simulink subsystem "YawController_SubSystem"  (R2021a)
settings: Solver=VariableStepAuto  StartTime=0.0  StopTime=10.0  RelTol=1e-3
undefined symbols (not defined in the file): DiscIntNeverNeededParam, drv, Ts, yaw_Ki, yaw_Kp
settings Model: Creator=utente-A  LastModifiedBy=utente-A

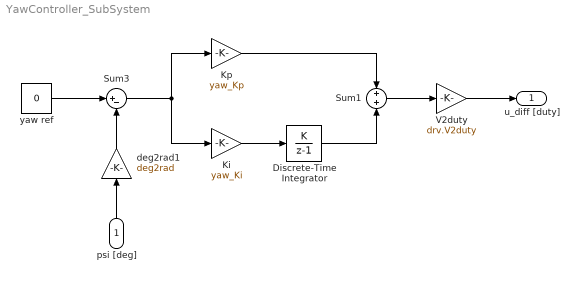
== system YawController_SubSystem ==
  psi [deg] : Inport
  Discrete-Time Integrator : DiscreteIntegrator  IntegratorMethod=Accumulation: Forward Euler  SampleTime=Ts  ICPrevOutput=DiscIntNeverNeededParam  ICPrevScaledInput=DiscIntNeverNeededParam
  Ki : Gain  Gain=yaw_Ki
  Kp : Gain  Gain=yaw_Kp
  Sum1 : Sum
  Sum3 : Sum  Inputs=|+-
  V2duty : Gain  Gain=drv.V2duty
  deg2rad1 : Gain  Gain=deg2rad
  yaw ref : Constant  Value=0
  u_diff [duty] : Outport
  wires:
  Sum3/1 -> Kp/1, Ki/1
  psi [deg]/1 -> deg2rad1/1
  deg2rad1/1 -> Sum3/2
  Ki/1 -> Discrete-Time Integrator/1
  Kp/1 -> Sum1/1
  Discrete-Time Integrator/1 -> Sum1/2
  Sum1/1 -> V2duty/1
  V2duty/1 -> u_diff [duty]/1
  yaw ref/1 -> Sum3/1
